simulink model "sim_tutorial3"  (Simulink 10.0)
settings: Solver=ode23tb  StartTime=0.0  StopTime=1.5  RelTol=1e-2  EnableMultiTasking=on
undefined symbols (not defined in the file): a, B, c, D
libraries: simulink3 x1
settings Model: Creator=bhisma  LastModifiedBy=bhisma  ExtModeTrigMode=oneshot  ExtModeArmWhenConnect=off
settings DataIOCC: SignalLoggingSaveFormat=ModelDataLogs
settings OptimizationCC: BlockReduction=off  BooleanDataType=off  LifeSpan=auto
settings DebuggingCC: SaveWithParameterizedLinksMsg=none  SignalResolutionControl=TryResolveAllWithWarning  MultiTaskDSMMsg=warning  MultiTaskCondExecSysMsg=none  SFUnexpectedBacktrackingDiag=error  SFNoUnconditionalDefaultTransitionDiag=error  SFExecutionAtInitializationDiag=warning  ArithmeticOperatorsInVariantConditions=error
settings HardwareCC: ProdBitPerPointer=64  ProdBitPerSizeT=64  ProdBitPerPtrDiffT=64  ProdLargestAtomicFloat=Float  ProdIntDivRoundTo=Zero  ProdEndianess=LittleEndian  ProdWordSize=64  ProdHWDeviceType=Intel->x86-64 (Windows64)  TargetUnknown=on
settings SFSimCC: SimUseLocalCustomCode=on  CustomCodeUndefinedFunction=FilterOut
settings RTWCC: RTWUseLocalCustomCode=on
settings CodeAppCC: StateflowObjectComments=off
settings GRTTargetCC: TargetLangStandard=C99 (ISO)
settings ConfigComp: CovMetricSettings=dwe  CovHtmlReporting=off  CovSaveCumulativeToWorkspaceVar=off  CovSaveSingleToWorkspaceVar=off

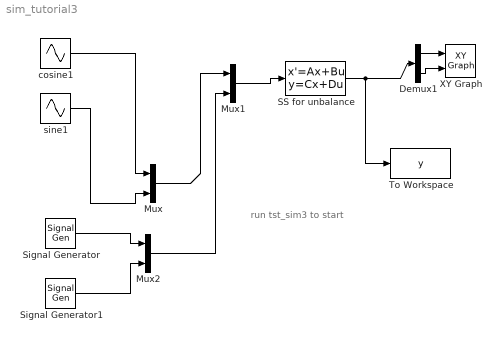
== system sim_tutorial3 ==
  note: run
      | tst_sim3
      | to start
  Demux1 : Demux  Outputs=2
  Mux : Mux  Inputs=2
  Mux1 : Mux  Inputs=2
  Mux2 : Mux  Inputs=2
  SS for unbalance : StateSpace  A=a  B=B  C=c  D=D  InitialCondition=0
  Signal Generator : SignalGenerator  WaveForm=square
  Signal Generator1 : SignalGenerator  WaveForm=square  Frequency=.9
  To Workspace : ToWorkspace  VariableName=y  SaveFormat=Structure With Time  SampleTime=-1
  XY Graph : simulink3/Sinks/XY Graph  xmin=-3e-6  xmax=3e-6  ymin=-3e-6  ymax=3e-6  st=-1
      settings: SourceProductName=Simulink  SourceProductBaseCode=SL
  cosine1 : Sin  Frequency=1.21  Phase=pi/2  SampleTime=0
  sine1 : Sin  SampleTime=0
  wires:
  Demux1/2 -> XY Graph/2
  Demux1/1 -> XY Graph/1
  sine1/1 -> Mux/2
  cosine1/1 -> Mux/1
  Mux1/1 -> SS for unbalance/1
  Mux/1 -> Mux1/1
  Signal Generator/1 -> Mux2/1
  Signal Generator1/1 -> Mux2/2
  Mux2/1 -> Mux1/2
  SS for unbalance/1 -> Demux1/1, To Workspace/1
